simulink model "LRC"  (Simulink 7.5)
settings: Solver=ode45  StartTime=0.0  StopTime=1e-3  RelTol=1e-3
settings Model: Creator=Liu zhiwei  LastModifiedBy=Liu zhiwei

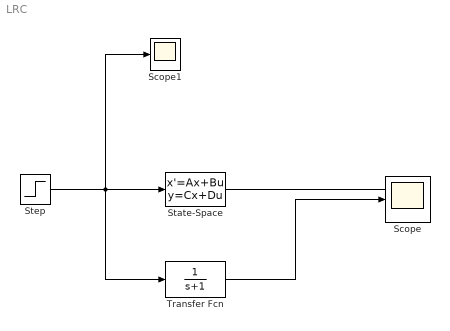
== system LRC ==
  Scope : Scope
  Scope1 : Scope
  State-Space : StateSpace
  Step : Step  Time=2e-4  After=2  SampleTime=0
  Transfer Fcn : TransferFcn  Denominator=[1 1]
  wires:
  Step/1 -> State-Space/1, Transfer Fcn/1, Scope1/1
  Transfer Fcn/1 -> Scope/1
  State-Space/1 -> ?
